simulink model "auv"  (R2022b)
settings: Solver=VariableStepAuto  StartTime=0.0  StopTime=50  FixedStep=0.000025  RelTol=1e-3
InitFcn:
  | param
StopFcn:
  | smoothing
  | dataplot
values from neighbouring files (symbols this model uses):
  C_lq = 1.18    [param.m]
  C_lu = 17.24    [param.m]
  C_lw = 38.06    [param.m]
  C_qq = 7.51    [param.m]
  C_qu = 106.03    [param.m]
  C_qw = 84.1    [param.m]
  D1 = 300    [param.m]
  I = 5.98    [param.m]
  m = 115    [param.m]
  P_init = eye(6)    [param.m]
  particles_init = mvnrnd(xi0, P0, N)    [param.m]
  q_hat_init = 0    [param.m]
  sample_time = min([T_z T_theta T_db])    [param.m]
  T_db = 1/freq_db    (= 0.025)    [param.m]
  T_theta = 1/freq_theta    (= 0.02)    [param.m]
  T_z = 1/freq_z    (= 0.0333333333333)    [param.m]
  theta_hat_init = pi/8*rand(1,1)    [param.m]
  u_hat_init = 0    [param.m]
  var_v_db = 0.2    [param.m]
  var_v_theta = 0.1    [param.m]
  var_v_z = 0.4    [param.m]
  var_w_q = 0.05    [param.m]
  var_w_u = 0.1    [param.m]
  var_w_w = 0.1    [param.m]
  w_hat_init = 0    [param.m]
  weights_init = 1/N*ones(N,1)    [param.m]
  x_hat_init = 140+20*rand(1,1)    [param.m]
  z_hat_init = 20+10*rand(1,1)    [param.m]
settings Model: Creator=Giovanni  LastModifiedBy=giopa

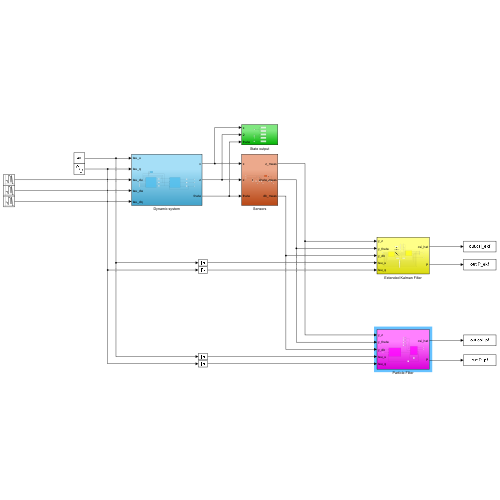
[thumbnail: Simulink's stored preview of the top-level diagram]
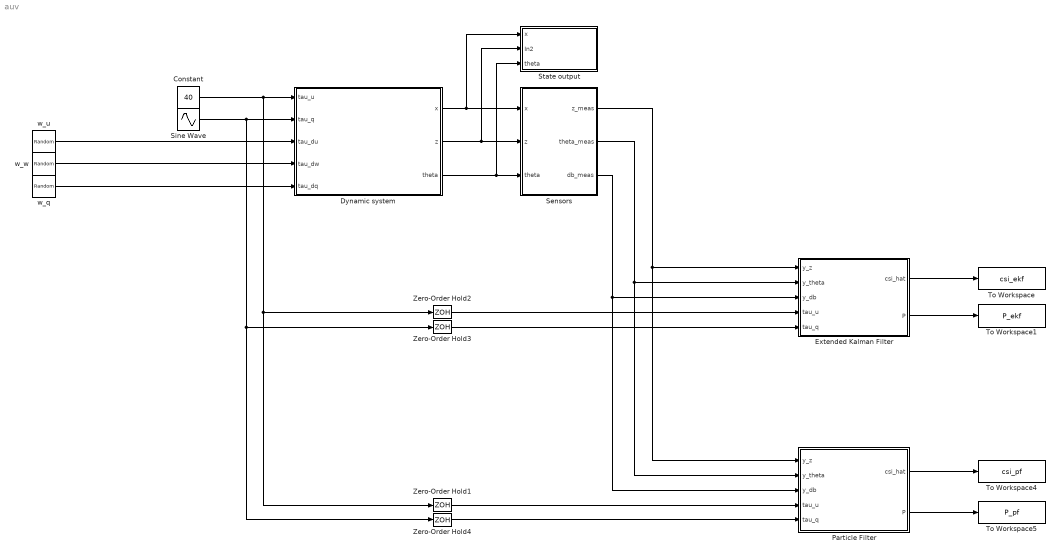
== system auv ==
  Constant : Constant  Value=40
  Dynamic system : Subsystem
  Extended Kalman Filter : Subsystem
  Particle Filter : Subsystem
  Sensors : Subsystem
  Sine Wave : Sin  Amplitude=2.2  Frequency=0.1969  SampleTime=0
  State output : Subsystem
  To Workspace : ToWorkspace  VariableName=csi_ekf  SaveFormat=Timeseries  SampleTime=-1
  To Workspace1 : ToWorkspace  VariableName=P_ekf  SaveFormat=Timeseries  SampleTime=-1
  To Workspace4 : ToWorkspace  VariableName=csi_pf  SaveFormat=Timeseries  SampleTime=-1
  To Workspace5 : ToWorkspace  VariableName=P_pf  SaveFormat=Timeseries  SampleTime=-1
  Zero-Order Hold{1..4} (4 alike) : ZeroOrderHold  SampleTime=sample_time
  w_q : RandomNumber  Variance=var_w_q  SampleTime=0.1
  w_u : RandomNumber  Variance=var_w_u  SampleTime=0.1
  w_w : RandomNumber  Variance=var_w_w  SampleTime=0.1
  wires:
  Constant/1 -> Zero-Order Hold1/1, Zero-Order Hold2/1, Dynamic system/1(tau_u)
  Sine Wave/1 -> Zero-Order Hold3/1, Zero-Order Hold4/1, Dynamic system/2(tau_q)
  w_u/1 -> Dynamic system/3(tau_du)
  w_w/1 -> Dynamic system/4(tau_dw)
  Dynamic system/3(theta) -> Sensors/3(theta), State output/3(theta)
  Sensors/1(z_meas) -> Extended Kalman Filter/1(y_z), Particle Filter/1(y_z)
  Sensors/2(theta_meas) -> Extended Kalman Filter/2(y_theta), Particle Filter/2(y_theta)
  Sensors/3(db_meas) -> Extended Kalman Filter/3(y_db), Particle Filter/3(y_db)
  w_q/1 -> Dynamic system/5(tau_dq)
  Extended Kalman Filter/1(csi_hat) -> To Workspace/1
  Extended Kalman Filter/2(P) -> To Workspace1/1
  Particle Filter/1(csi_hat) -> To Workspace4/1
  Particle Filter/2(P) -> To Workspace5/1
  Zero-Order Hold4/1 -> Particle Filter/5(tau_q)
  Zero-Order Hold1/1 -> Particle Filter/4(tau_u)
  Dynamic system/1(x) -> Sensors/1(x), State output/1(x)
  Dynamic system/2(z) -> Sensors/2(z), State output/2(In2)
  Zero-Order Hold2/1 -> Extended Kalman Filter/4(tau_u)
  Zero-Order Hold3/1 -> Extended Kalman Filter/5(tau_q)

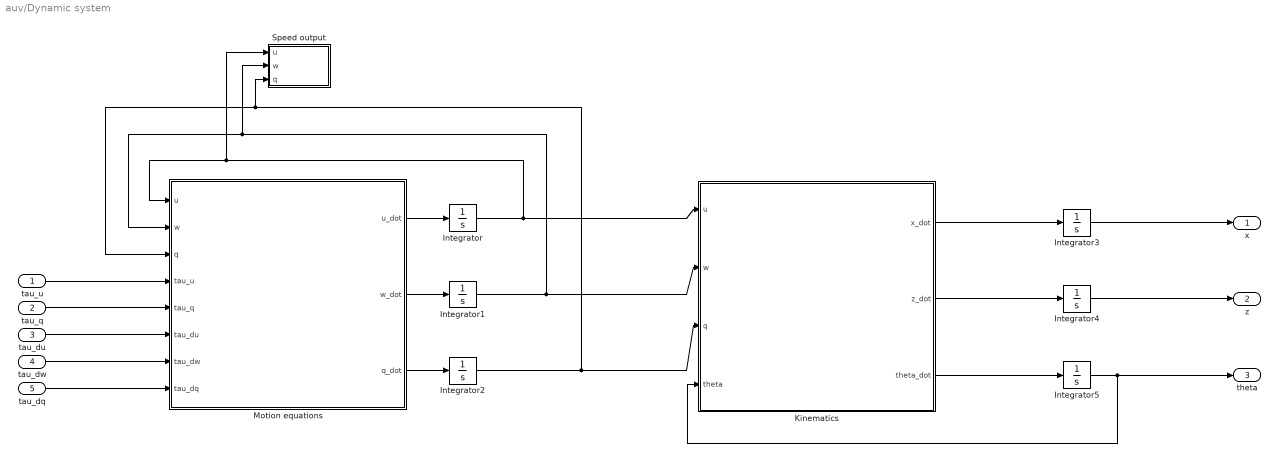
== system auv/Dynamic system ==
  tau_u : Inport
  tau_q : Inport  Port=2
  tau_du : Inport  Port=3
  tau_dw : Inport  Port=4
  tau_dq : Inport  Port=5
  Integrator{,1..2,5} (4 alike) : Integrator
  Integrator3 : Integrator  InitialCondition=150
  Integrator4 : Integrator  InitialCondition=25
  Kinematics : MATLAB Function  TreatAsAtomicUnit=on
  Motion equations : MATLAB Function  TreatAsAtomicUnit=on
  Speed output : Subsystem
  x : Outport
  z : Outport  Port=2
  theta : Outport  Port=3
  wires:
  Integrator3/1 -> x/1
  Kinematics/2(z_dot) -> Integrator4/1
  Integrator/1 -> Motion equations/1(u), Speed output/1(u), Kinematics/1(u)
  tau_du/1 -> Motion equations/6(tau_du)
  Integrator1/1 -> Motion equations/2(w), Speed output/2(w), Kinematics/2(w)
  Motion equations/2(w_dot) -> Integrator1/1
  tau_u/1 -> Motion equations/4(tau_u)
  Integrator5/1 -> theta/1, Kinematics/4(theta)
  Motion equations/1(u_dot) -> Integrator/1
  Motion equations/3(q_dot) -> Integrator2/1
  Integrator2/1 -> Motion equations/3(q), Speed output/3(q), Kinematics/3(q)
  Kinematics/3(theta_dot) -> Integrator5/1
  Kinematics/1(x_dot) -> Integrator3/1
  tau_q/1 -> Motion equations/5(tau_q)
  Integrator4/1 -> z/1
  tau_dw/1 -> Motion equations/7(tau_dw)
  tau_dq/1 -> Motion equations/8(tau_dq)

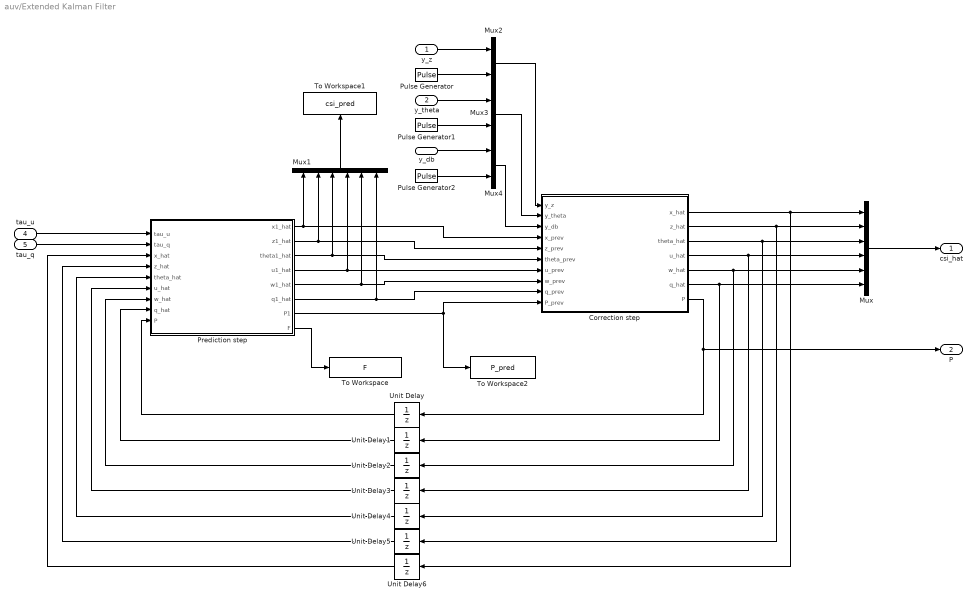
== system auv/Extended Kalman Filter ==
  y_z : Inport
  y_theta : Inport  Port=2
  y_db : Inport  Port=3
  tau_u : Inport  Port=4
  tau_q : Inport  Port=5
  Correction step : MATLAB Function  TreatAsAtomicUnit=on  SystemSampleTime=sample_time
  Mux : Mux  Inputs=6
  Mux1 : Mux  Inputs=6
  Mux2 : Mux  Inputs=2
  Mux3 : Mux  Inputs=2
  Mux4 : Mux  Inputs=2
  Prediction step : MATLAB Function  TreatAsAtomicUnit=on  SystemSampleTime=sample_time
  Pulse Generator : DiscretePulseGenerator  PulseType=Time based  Period=T_z  PulseWidth=10
  Pulse Generator1 : DiscretePulseGenerator  PulseType=Time based  Period=T_theta  PulseWidth=10
  Pulse Generator2 : DiscretePulseGenerator  PulseType=Time based  Period=T_db  PulseWidth=10
  To Workspace : ToWorkspace  VariableName=F  SaveFormat=Timeseries  SampleTime=-1
  To Workspace1 : ToWorkspace  VariableName=csi_pred  SaveFormat=Timeseries  SampleTime=-1
  To Workspace2 : ToWorkspace  VariableName=P_pred  SaveFormat=Timeseries  SampleTime=-1
  Unit Delay : UnitDelay  InitialCondition=P_init  SampleTime=-1  HasFrameUpgradeWarning=on
  Unit Delay1 : UnitDelay  InitialCondition=q_hat_init  SampleTime=-1  HasFrameUpgradeWarning=on
  Unit Delay2 : UnitDelay  InitialCondition=w_hat_init  SampleTime=-1  HasFrameUpgradeWarning=on
  Unit Delay3 : UnitDelay  InitialCondition=u_hat_init  SampleTime=-1  HasFrameUpgradeWarning=on
  Unit Delay4 : UnitDelay  InitialCondition=theta_hat_init  SampleTime=-1  HasFrameUpgradeWarning=on
  Unit Delay5 : UnitDelay  InitialCondition=z_hat_init  SampleTime=-1  HasFrameUpgradeWarning=on
  Unit Delay6 : UnitDelay  InitialCondition=x_hat_init  SampleTime=-1  HasFrameUpgradeWarning=on
  csi_hat : Outport
  P : Outport  Port=2
  wires:
  Correction step/2(z_hat) -> Unit Delay5/1, Mux/2
  Prediction step/7(P1) -> Correction step/10(P_prev), To Workspace2/1
  Correction step/7(P) -> Unit Delay/1, P/1
  Unit Delay6/1 -> Prediction step/3(x_hat)
  tau_q/1 -> Prediction step/2(tau_q)
  Unit Delay2/1 -> Prediction step/7(w_hat)
  Correction step/3(theta_hat) -> Unit Delay4/1, Mux/3
  Unit Delay3/1 -> Prediction step/6(u_hat)
  Correction step/5(w_hat) -> Unit Delay2/1, Mux/5
  Prediction step/8(F) -> To Workspace/1
  Unit Delay5/1 -> Prediction step/4(z_hat)
  Correction step/6(q_hat) -> Unit Delay1/1, Mux/6
  Correction step/4(u_hat) -> Unit Delay3/1, Mux/4
  Unit Delay1/1 -> Prediction step/8(q_hat)
  Prediction step/3(theta1_hat) -> Correction step/6(theta_prev), Mux1/3
  tau_u/1 -> Prediction step/1(tau_u)
  Prediction step/6(q1_hat) -> Correction step/9(q_prev), Mux1/6
  Prediction step/1(x1_hat) -> Correction step/4(x_prev), Mux1/1
  Prediction step/2(z1_hat) -> Correction step/5(z_prev), Mux1/2
  Prediction step/5(w1_hat) -> Correction step/8(w_prev), Mux1/5
  Unit Delay4/1 -> Prediction step/5(theta_hat)
  Prediction step/4(u1_hat) -> Correction step/7(u_prev), Mux1/4
  Unit Delay/1 -> Prediction step/9(P)
  Correction step/1(x_hat) -> Unit Delay6/1, Mux/1
  Mux/1 -> csi_hat/1
  Mux1/1 -> To Workspace1/1
  y_z/1 -> Mux2/1
  Pulse Generator/1 -> Mux2/2
  y_theta/1 -> Mux3/1
  Pulse Generator1/1 -> Mux3/2
  y_db/1 -> Mux4/1
  Pulse Generator2/1 -> Mux4/2
  Mux2/1 -> Correction step/1(y_z)
  Mux3/1 -> Correction step/2(y_theta)
  Mux4/1 -> Correction step/3(y_db)

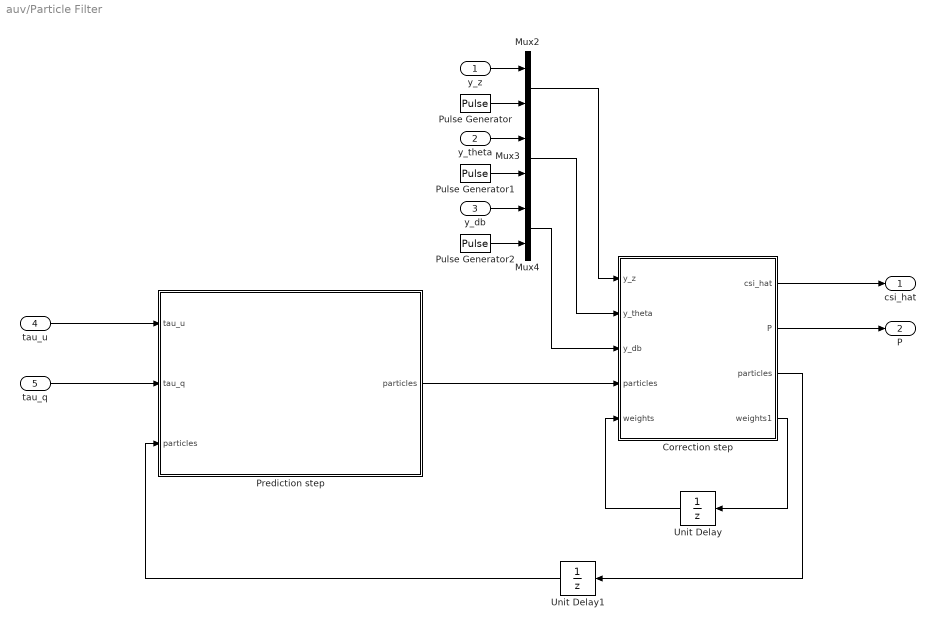
== system auv/Particle Filter ==
  y_z : Inport
  y_theta : Inport  Port=2
  y_db : Inport  Port=3
  tau_u : Inport  Port=4
  tau_q : Inport  Port=5
  Correction step : MATLAB Function  TreatAsAtomicUnit=on  SystemSampleTime=sample_time
  Mux2 : Mux  Inputs=2
  Mux3 : Mux  Inputs=2
  Mux4 : Mux  Inputs=2
  Prediction step : MATLAB Function  TreatAsAtomicUnit=on  SystemSampleTime=sample_time
  Pulse Generator : DiscretePulseGenerator  PulseType=Time based  Period=T_z  PulseWidth=10
  Pulse Generator1 : DiscretePulseGenerator  PulseType=Time based  Period=T_theta  PulseWidth=10
  Pulse Generator2 : DiscretePulseGenerator  PulseType=Time based  Period=T_db  PulseWidth=10
  Unit Delay : UnitDelay  InitialCondition=weights_init  SampleTime=-1  HasFrameUpgradeWarning=on
  Unit Delay1 : UnitDelay  InitialCondition=particles_init  SampleTime=-1  HasFrameUpgradeWarning=on
  csi_hat : Outport
  P : Outport  Port=2
  wires:
  tau_q/1 -> Prediction step/2(tau_q)
  Correction step/4(weights1) -> Unit Delay/1
  Correction step/3(particles) -> Unit Delay1/1
  Prediction step/1(particles) -> Correction step/4("particles ")
  Unit Delay/1 -> Correction step/5(weights)
  Unit Delay1/1 -> Prediction step/3("particles ")
  Correction step/1(csi_hat) -> csi_hat/1
  tau_u/1 -> Prediction step/1(tau_u)
  Correction step/2(P) -> P/1
  Pulse Generator2/1 -> Mux4/2
  y_theta/1 -> Mux3/1
  Pulse Generator1/1 -> Mux3/2
  Pulse Generator/1 -> Mux2/2
  y_z/1 -> Mux2/1
  Mux2/1 -> Correction step/1(y_z)
  Mux4/1 -> Correction step/3(y_db)
  y_db/1 -> Mux4/1
  Mux3/1 -> Correction step/2(y_theta)

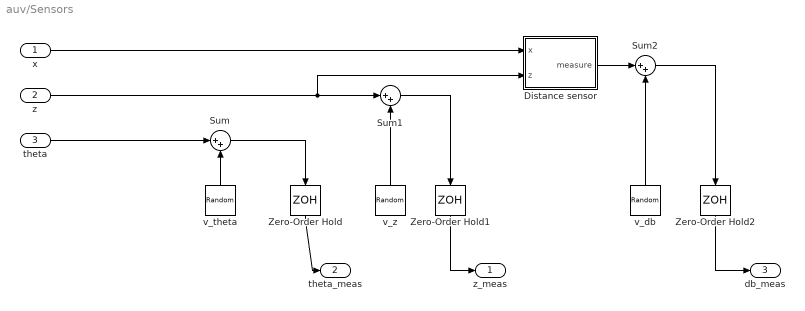
== system auv/Sensors ==
  x : Inport
  z : Inport  Port=2
  theta : Inport  Port=3
  Distance sensor : MATLAB Function  TreatAsAtomicUnit=on
  Sum : Sum  Inputs=|++
  Sum1 : Sum  Inputs=|++
  Sum2 : Sum  Inputs=|++
  Zero-Order Hold : ZeroOrderHold  SampleTime=T_theta
  Zero-Order Hold1 : ZeroOrderHold  SampleTime=T_z
  Zero-Order Hold2 : ZeroOrderHold  SampleTime=T_db
  v_db : RandomNumber  Variance=var_v_db  SampleTime=T_db
  v_theta : RandomNumber  Variance=var_v_theta  SampleTime=T_theta
  v_z : RandomNumber  Variance=var_v_z  SampleTime=T_z
  z_meas : Outport
  theta_meas : Outport  Port=2
  db_meas : Outport  Port=3
  wires:
  v_db/1 -> Sum2/2
  z/1 -> Sum1/1, Distance sensor/2(z)
  Sum/1 -> Zero-Order Hold/1
  v_z/1 -> Sum1/2
  Distance sensor/1(measure) -> Sum2/1
  Sum1/1 -> Zero-Order Hold1/1
  v_theta/1 -> Sum/2
  theta/1 -> Sum/1
  x/1 -> Distance sensor/1(x)
  Sum2/1 -> Zero-Order Hold2/1
  Zero-Order Hold1/1 -> z_meas/1
  Zero-Order Hold2/1 -> db_meas/1
  Zero-Order Hold/1 -> theta_meas/1

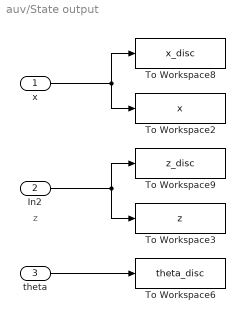
== system auv/State output ==
  note: z
  x : Inport
  In2 : Inport  Port=2
  theta : Inport  Port=3
  To Workspace2 : ToWorkspace  VariableName=x  SaveFormat=Timeseries  SampleTime=-1
  To Workspace3 : ToWorkspace  VariableName=z  SaveFormat=Timeseries  SampleTime=-1
  To Workspace6 : ToWorkspace  VariableName=theta_disc  SaveFormat=Timeseries  SampleTime=sample_time
  To Workspace8 : ToWorkspace  VariableName=x_disc  SaveFormat=Timeseries  SampleTime=sample_time
  To Workspace9 : ToWorkspace  VariableName=z_disc  SaveFormat=Timeseries  SampleTime=sample_time
  wires:
  x/1 -> To Workspace8/1, To Workspace2/1
  In2/1 -> To Workspace3/1, To Workspace9/1
  theta/1 -> To Workspace6/1

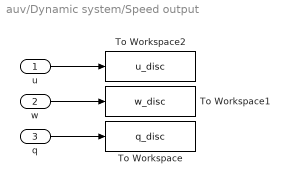
== system auv/Dynamic system/Speed output ==
  u : Inport
  w : Inport  Port=2
  q : Inport  Port=3
  To Workspace : ToWorkspace  VariableName=q_disc  SaveFormat=Timeseries  SampleTime=sample_time
  To Workspace1 : ToWorkspace  VariableName=w_disc  SaveFormat=Timeseries  SampleTime=sample_time
  To Workspace2 : ToWorkspace  VariableName=u_disc  SaveFormat=Timeseries  SampleTime=sample_time
  wires:
  u/1 -> To Workspace2/1
  w/1 -> To Workspace1/1
  q/1 -> To Workspace/1

== matlab function auv/Extended Kalman Filter/Correction step ==
  data: y_z input; x_hat output; y_theta input; y_db input; x_prev input; z_prev input; theta_prev input; u_prev input; w_prev input; q_prev input; P_prev input; z_hat output; theta_hat output; u_hat output; w_hat output; q_hat output; P output; D1 parameter; var_v_db parameter; var_v_theta parameter; var_v_z parameter
function [x_hat,z_hat,theta_hat,u_hat,w_hat,q_hat,P] = correct_ekf(y_z,y_theta,y_db,x_prev,z_prev,theta_prev,u_prev,w_prev,q_prev,P_prev,D1,var_v_db,var_v_theta,var_v_z)

%% Gestione delle misure dei sensori e inizializzazione
    % pulse = 1 -> arriva una nuova misura del sensore
    % pulse = 0 -> non c'è nessuna nuova misura
    
    % Misure sensori
    meas_z = y_z(1,:);                                % misura profondità z
    meas_theta = y_theta(1,:);                        % misura angolo beccheggio theta
    meas_db = y_db(1,:);                              % misura distanza db 

    pulse_z = y_z(2,:);                               % impulso profondimetro
    pulse_theta = y_theta(2,:);                       % impulso giroscopio
    pulse_db = y_db(2,:);                             % impulso sensore di distanza

    % Inizializzo le variabili utilizzate nei calcoli
    % N.B. dimensione variabile sulla base di quante nuove misure ricevo

    % Jacobiani del modello di misura rispetto allo stato e ai rumori
    H = zeros(pulse_z+pulse_theta+pulse_db,6);                
    M = eye(pulse_z+pulse_theta+pulse_db);
    % Digonale matrice di covarianza dei rumori sulle misure
    R_vec = zeros(pulse_z+pulse_theta+pulse_db,1);             
    
    % Stato predetto in ingresso
    xi_prev = [x_prev z_prev theta_prev u_prev w_prev q_prev]';
    % Inizializzazione innovazione
    e = zeros(pulse_z+pulse_theta+pulse_db,1);                

%% Inserisco i valori corrispondenti alle misure disponibili

    % Se la misura per z è disponibile, la corrispondente riga del
    % jacobiano è la prima, per i vettori è il primo elemento.

    if pulse_z == 1                                            
        H(1,:) = [0 1 0 0 0 0];                                 
        R_vec(1) = var_v_z;
        e(1) = meas_z - z_prev;
    end
    
    % Se le misure per z e theta sono entrambe disponibili, i dati relativi
    % a theta sono posizionati nella seconda riga. Se è disponibile solo
    % theta allora i dati sono posizionati nella prima riga. Ugualmente per
    % i vettori.

    if pulse_theta == 1                                        
        H(pulse_z+pulse_theta,:) = [0 0 1 0 0 0];               
        R_vec(pulse_z+pulse_theta) = var_v_theta;          
        e(pulse_z+pulse_theta) = wrapToPi(meas_theta - theta_prev);
    end

    % Come sopra, per db

    if pulse_db == 1                                           
        H(pulse_z+pulse_theta+pulse_db,:) = [-(D1-x_prev)/sqrt((D1-x_prev)^2+z_prev^2) z_prev/sqrt((D1-x_prev)^2+z_prev^2) 0 0 0 0];
        R_vec(pulse_z+pulse_theta+pulse_db) = var_v_db;
        e(pulse_z+pulse_theta+pulse_db) = meas_db - sqrt((D1-x_prev)^2+z_prev^2);
    end

%% Applico la correzione
    R = diag(R_vec);                  % Matrice covarianza disturbo sensori
    S = H*P_prev*H' + M*R*M';         % Matrice covarianza innovazione     
    L = P_prev*H'/S;                  % Guadagno correzione
    
    % Stato corretto ->  X_k|k
    xi_hat = xi_prev + L*e;  
    % Matrice di covarianza associata alla stima -> P_k|k 
    P = (eye(6) - L*H)*P_prev*(eye(6) - L*H)' + L*M*R*M'*L';   
    
%% Output blocco di correzione 
    x_hat = xi_hat(1);
    z_hat = xi_hat(2);
    theta_hat = xi_hat(3);
    u_hat = xi_hat(4);
    w_hat = xi_hat(5);
    q_hat = xi_hat(6);

end

== matlab function auv/Particle Filter/Prediction step ==
  data: particles output; tau_u input; tau_q input; particles input; var_w_u parameter; var_w_w parameter; var_w_q parameter; sample_time parameter; m parameter; C_qq parameter; C_lq parameter; C_qw parameter; C_lw parameter; C_qu parameter; C_lu parameter; I parameter
function particles = predict_pf(tau_u,tau_q,particles,var_w_u,var_w_w,var_w_q,sample_time,m,C_qq,C_lq,C_qw,C_lw,C_qu,C_lu,I)

    for i=1:size(particles,1)
    
        % Realizzazione di rumore coerente per una singola particella
        noise_u = sqrt(var_w_u)*randn(1,1);
        noise_w = sqrt(var_w_w)*randn(1,1);
        noise_q = sqrt(var_w_q)*randn(1,1);
    
        %% PREDIZIONE 
        % predizione -> applico il modello del processo f
        % STEP di predizione    X_k+1|k = f(X_k|k,...,W_k)  applico modello
        %                       W_k+1|k = W_k|k pesi invariati 
        particles(i,1) = particles(i,1) + sample_time*(particles(i,4)*cos(particles(i,3)) + particles(i,5)*sin(particles(i,3)));
        particles(i,2) = particles(i,2) + sample_time*(-particles(i,4)*sin(particles(i,3)) + particles(i,5)*cos(particles(i,3)));
        particles(i,3) = particles(i,3) + sample_time*particles(i,6);
        particles(i,4) = particles(i,4) + sample_time*(-m*particles(i,5)*particles(i,6) - C_lu*particles(i,4) - C_qu*abs(particles(i,4))*particles(i,4) + tau_u + noise_u)/m;
        particles(i,5) = particles(i,5) + sample_time*(m*particles(i,4)*particles(i,6) - C_lw*particles(i,5) - C_qw*abs(particles(i,5))*particles(i,5) + noise_w)/m;
        particles(i,6) = particles(i,6) + sample_time*(-C_lq*particles(i,6) - C_qq*abs(particles(i,6))*particles(i,6) + tau_q + noise_q)/I;
    
    end

end

== matlab function auv/Particle Filter/Correction step ==
  data: y_z input; y_theta input; y_db input; particles input; weights input; csi_hat output; P output; particles output; weights1 output; D1 parameter; var_v_theta parameter; var_v_db parameter; var_v_z parameter
function [csi_hat,P,particles,weights1] = correct_pf(y_z,y_theta,y_db,particles,weights,D1,var_v_theta,var_v_db,var_v_z)
    
    % Si ricava la deviazione standard dalla varianza, per utilizzarla
    % nella funzione normpdf
    sigma_z = sqrt(var_v_z);
    sigma_theta = sqrt(var_v_theta);
    sigma_db = sqrt(var_v_db);

%% Misure | Impulsi sensori
    meas_z = y_z(1,:);
    meas_theta = y_theta(1,:);
    meas_db = y_db(1,:);

    pulse_z = y_z(2,:);
    pulse_theta = y_theta(2,:);
    pulse_db = y_db(2,:);

%% Parametri per il ricampionamento     
    threshold = 0.8;        % Frequenza ricampionamento: 1 -> sempre, 0 -> mai
    eps = 0.0055;           % Disturbo per la generazione di nuovi campioni -> distribuisce
                            % le particelle per evitare che ce se siano di uguali

%% Calcolo della verosimiglianza
    % Essendo un prodotto, se la misura è disponibile (pulse = 1) allora viene
    % calcolata la verosimiglianza, altrimenti assumerà valore 1

    % Inizializzazione likelihood per le singole misure
    l_z = ones(size(particles,1),1);
    l_theta = ones(size(particles,1),1);
    l_db = ones(size(particles,1),1);
    
    if pulse_z == 1
        for i=1:size(particles,1)
            l_z(i) = normpdf(meas_z-particles(i,2),0,sigma_z);
        end
    end

    if pulse_theta == 1
        for i=1:size(particles,1)
            l_theta(i) = normpdf(wrapToPi(meas_theta-particles(i,3)),0,sigma_theta);
        end
    end

    if pulse_db == 1
        for i=1:size(particles,1)
            l_db(i) = normpdf(meas_db-sqrt((D1-particles(i,1))^2+particles(i,2)^2),0,sigma_db);
        end
    end

    likelihood = l_z.*l_theta.*l_db;                       
    % Nuovi pesi come pesi a priori per la likelihood, poi normalizzo
    weights1 = (weights.*likelihood)/sum(weights.*likelihood);
    

%% Ricampionamento
    N_eff = 1/sum((weights1).^2);                    % Numero efficace di particelle
    
    % 0     S1          S2...    1  sommatoria s=1
    % |-----|------------|-------|
    %   w1      w2          w..   
    % a estratto tra 0 e 1 uniformemente, a apparterrà ad uno dei segmenti
    % Si; è più probabile estrarre in corrispondenza di un segmento più
    % "ampio" i.e. peso più alto -> rigenero più campioni in corrispondenza
    % del segmento (e quindi particella) con peso più alto

    if N_eff/size(particles,1) <= threshold          % Entro nel ciclo se sotto la soglia 
        s = cumsum(weights1);
        new_particles = zeros(size(particles));
        for j = 1:size(particles,1)
            a = rand(1);
            dist = eps*randn(6,1);

            % Rigenero i campioni con probabilità definita dai pesi e li
            % perturbo per evitare impoverimento
            i = find(s>=a,1);
            new_particles(j,:) = particles(i,:) + dist';
        end
        % Ricalcolo i pesi distribuendoli uniformemente tra le particelle ricampionate
        new_weights = 1/size(weights1,1)*ones(size(weights,1),1); 
        % Aggiorno le variabili
        particles = new_particles;
        weights1 = new_weights;
    end
   
%% Calcolo della stima dello stato come media pesata delle particelle
    csi_hat = particles'*weights1;

    % Matrice di covarianza associata alla stima
    P = zeros(6,6);
    for i=1:size(particles,1)
        P = P + weights1(i)*(particles(i,:)' - csi_hat)*(particles(i,:)' - csi_hat)';
    end

end

== matlab function auv/Dynamic system/Kinematics ==
  settings: updateMethod=CONTINUOUS
  data: u input; x_dot output; w input; q input; theta input; z_dot output; theta_dot output
function [x_dot, z_dot, theta_dot] = kinematics(u,w,q,theta)

 %% DEFINISCO PARAMETRI USATI NELLA FUNZIONE
    Rz = [cos(theta) sin(theta) 0   ; %
         -sin(theta) cos(theta) 0   ; % MATRICE DI ROTAZIONE ATTORNO ALL'ASSE Z
            0           0       1 ] ; % 
%% CAMBIO SISTEMA DI RIFERIMENTO DA TERNA BODY A SISTEMA FISSO     
    out = Rz*[u w q]';

%% FORNISCO IN USCITA LE SINGOLE COMPONENTI    
    x_dot     = out(1);
    z_dot     = out(2);
    theta_dot = out(3);

== matlab function auv/Dynamic system/Motion equations ==
  settings: updateMethod=CONTINUOUS
  data: u input; u_dot output; w input; q input; tau_u input; tau_q input; tau_du input; tau_dw input; tau_dq input; w_dot output; q_dot output; m parameter; I parameter; C_qu parameter; C_lu parameter; C_lw parameter; C_qw parameter; C_lq parameter; C_qq parameter
function [u_dot,w_dot,q_dot] = motion(u,w,q,tau_u,tau_q,tau_du,tau_dw,tau_dq,m, I, C_qu, C_lu, C_lw, C_qw, C_lq, C_qq)

 % Inversione della dinamica del sistema per ricavare le accelerazioni,
 % portiamo le informazioni in forma matriciale per semplicità
    
    U = [u w q]';                               % Vettore velocità

    B = [m 0 0 ;
         0 m 0 ;                                % Matrice inerzia
         0 0 I];

    C = [  0     0   m*w ;                      %
           0     0  -m*u ;                      % Matrice coriolis
         -m*w   m*u   0 ];                      %

    F = [ C_lu+C_qu*abs(u)   0            0              ;  %
              0          C_lw+C_qw*abs(w) 0              ;  %   Matrice reistenza avanzamento
              0              0       C_lq + C_qq*abs(q) ];  %

    Q = [tau_u 0 tau_q]';                       % Vettore controllo
    D = [tau_du tau_dw tau_dq]';                % Vettore disturbo
    
    O = B\(Q+D-C*U-F*U);                        % Inversione dinamica 
    
    u_dot=O(1);                                 
    w_dot=O(2);
    q_dot=O(3);

end

== matlab function auv/Sensors/Distance sensor ==
  data: x input; measure output; z input; D1 parameter
function measure = sens(x,z,D1)

    measure = sqrt((D1-x)^2+z^2);

end

== matlab function auv/Extended Kalman Filter/Prediction step ==
  data: tau_u input; tau_q input; x_hat input; x1_hat output; z_hat input; theta_hat input; u_hat input; w_hat input; q_hat input; P input; z1_hat output; theta1_hat output; u1_hat output; w1_hat output; q1_hat output; P1 output; F output; I parameter; m parameter; C_qq parameter; C_lq parameter; C_qw parameter; C_lw parameter; C_qu parameter; C_lu parameter; var_w_u parameter; var_w_q parameter; var_w_w parameter; sample_time parameter
function [x1_hat,z1_hat,theta1_hat,u1_hat,w1_hat,q1_hat,P1,F] = predict_ekf(tau_u,tau_q,x_hat,z_hat,theta_hat,u_hat,w_hat,q_hat,P,I,m,C_qq,C_lq,C_qw,C_lw,C_qu,C_lu,var_w_u,var_w_q,var_w_w,sample_time)

    Q = [var_w_u 0 0;
         0 var_w_w 0;     % Covarianza del disturbo sugli ingressi               
         0 0 var_w_q];
    
%% PREDIZIONE
    %  X_k+1 = X_k + dt * X_dot
    %  predizione vettore di stato esteso 
    x1_hat = x_hat + sample_time*(u_hat*cos(theta_hat) + w_hat*sin(theta_hat));
    z1_hat = z_hat + sample_time*(-u_hat*sin(theta_hat) + w_hat*cos(theta_hat));
    theta1_hat = theta_hat + sample_time*q_hat;
    u1_hat = u_hat + sample_time*(-m*w_hat*q_hat - C_lu*u_hat - C_qu*abs(u_hat)*u_hat + tau_u)/m;
    w1_hat = w_hat + sample_time*(m*u_hat*q_hat - C_lw*w_hat - C_qw*abs(w_hat)*w_hat)/m;
    q1_hat = q_hat + sample_time*(-C_lq*q_hat - C_qq*abs(q_hat)*q_hat + tau_q)/I;
    
%% LINEARIZZAZIONE

    % F jacobiano del modello di processo f rispetto allo stato valutato
    % in x = x_pred k|k e Wk=0 
    F = [1 0 sample_time*(-u_hat*sin(theta_hat)+w_hat*cos(theta_hat)) sample_time*cos(theta_hat) sample_time*sin(theta_hat) 0;
         0 1 sample_time*(-u_hat*cos(theta_hat)-w_hat*sin(theta_hat)) sample_time*(-sin(theta_hat)) sample_time*cos(theta_hat) 0;
         0 0 1 0 0 sample_time;
         0 0 0 1+sample_time*(-C_lu-C_qu*(abs(u_hat)+u_hat*sign(u_hat)))/m  sample_time*(-q_hat) sample_time*(-w_hat);
         0 0 0 sample_time*q_hat 1+sample_time*(-C_lw-C_qw*(abs(w_hat)+w_hat*sign(w_hat)))/m  sample_time*u_hat;
         0 0 0 0 0 1+sample_time*(-C_lq-C_qq*(abs(q_hat)+q_hat*sign(q_hat)))/I];
    
    % D jacobiano del modello di processo rispetto ai disturbi valutato
    % nello stesso punto di linearizzazione
    D = [0 0 0;
         0 0 0;
         0 0 0;
         sample_time*1/m 0 0;
         0 sample_time*1/m 0;
         0 0 sample_time*1/I];
    
    % Covarianza della stima al passo k+1|k
    P1 = F*P*F' + D*Q*D';    

end
